simulink model "host_receive"  (R2015a)
settings: Solver=FixedStepDiscrete  StartTime=0.0  StopTime=inf  RelTol=1e-3
libraries: embdlinuxlib x2, simulink x1
settings Model: Creator=sbiagion  LastModifiedBy=sbiagion
settings DebuggingCC: UnderspecifiedInitializationDetection=Classic  MergeDetectMultiDrivingBlocksExec=none  SolverPrmCheckMsg=warning  MultiTaskRateTransMsg=warning

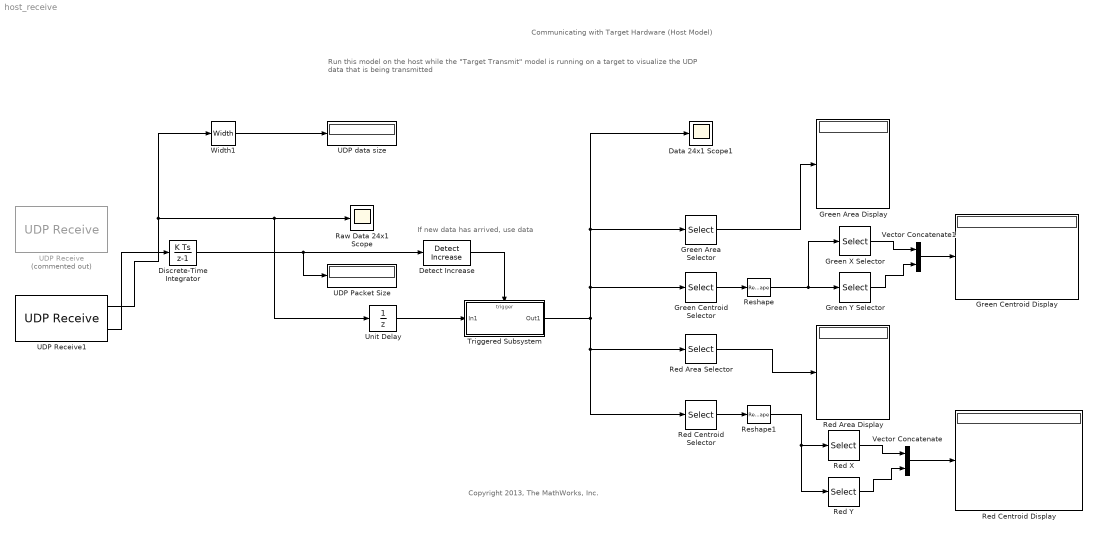
== system host_receive ==
  note: Run this model on the host while the "Target Transmit" model is running on a target to visualize the UDP data that is being transmitted
  note: Copyright 2013, The MathWorks, Inc.
  note: If new data has arrived, use data
  note: Communicating with Target Hardware
      | (Host Model)
  Data 24x1 Scope1 : Scope
      settings: ShowLegends=on  TimeRange=10  YMin=-100  YMax=1200  MaxDataPoints=100
  Detect Increase : simulink/Logic and Bit Operations/Detect Increase  vinit=0.0  InputProcessing=Inherited  OutDataTypeStr=boolean
  Discrete-Time Integrator : DiscreteIntegrator  gainval=1e4  SampleTime=-1
  Green Area Display : Display
  Green Area Selector : Selector  InputPortWidth=24  Indices=[1:4]
  Green Centroid Display : Display
  Green Centroid Selector : Selector  InputPortWidth=24  Indices=[5:12]
  Green X Selector : Selector  NumberOfDimensions=2  InputPortWidth=24  IndexOptions=Select all,Index vector (dialog)  Indices=[17:24],2  OutputSizes=1,1
  Green Y Selector : Selector  NumberOfDimensions=2  InputPortWidth=24  IndexOptions=Select all,Index vector (dialog)  Indices=[17:24],1  OutputSizes=1,1
  Raw Data 24x1 Scope : Scope
      settings: ShowLegends=on  TimeRange=10  YMin=-100  YMax=1200  MaxDataPoints=100
  Red Area Display : Display
  Red Area Selector : Selector  InputPortWidth=24  Indices=[13:16]
  Red Centroid Display : Display
  Red Centroid Selector : Selector  InputPortWidth=24  Indices=[17:24]
  Red X : Selector  NumberOfDimensions=2  InputPortWidth=24  IndexOptions=Select all,Index vector (dialog)  Indices=[17:24],2  OutputSizes=1,1
  Red Y : Selector  NumberOfDimensions=2  InputPortWidth=24  IndexOptions=Select all,Index vector (dialog)  Indices=[17:24],1  OutputSizes=1,1
  Reshape : Reshape  OutputDimensionality=Customize  OutputDimensions=[4,2]
  Reshape1 : Reshape  OutputDimensionality=Customize  OutputDimensions=[4,2]
  Triggered Subsystem : Subsystem  TreatAsAtomicUnit=on
  UDP Packet Size : Display
  UDP Receive : embdlinuxlib/UDP Receive  Commented=on  localURL='0.0.0.0'  localPort=25001  remoteURL='0.0.0.0'  remotePort=-1  recvBufferSize=8192  signalDatatype=int32  dims=24  isVarSize=off  showBlockingTime=off  blockingTime=0  sampletime=0.1  blockPlatform=BeagleBoard
  UDP Receive1 : embdlinuxlib/UDP Receive  localURL='0.0.0.0'  localPort=25000  remoteURL='0.0.0.0'  remotePort=-1  recvBufferSize=8192  signalDatatype=int32  dims=24  isVarSize=off  showBlockingTime=off  blockingTime=0  sampletime=0.1  blockPlatform=Raspberry Pi
  UDP data size : Display
  Unit Delay : UnitDelay  SampleTime=-1
  Vector Concatenate : Concatenate  Mode=Multidimensional array  ConcatenateDimension=2
  Vector Concatenate1 : Concatenate  Mode=Multidimensional array  ConcatenateDimension=2
  Width1 : Width
  wires:
  UDP Receive1/2 -> Discrete-Time Integrator/1
  Discrete-Time Integrator/1 -> UDP Packet Size/1, Detect Increase/1
  UDP Receive1/1 -> Width1/1, Unit Delay/1, Raw Data 24x1 Scope/1
  Width1/1 -> UDP data size/1
  Triggered Subsystem/1(Out1) -> Red Area Selector/1, Red Centroid Selector/1, Green Centroid Selector/1, Data 24x1 Scope1/1, Green Area Selector/1
  Detect Increase/1 -> Triggered Subsystem/Trigger
  Unit Delay/1 -> Triggered Subsystem/1(In1)
  Green Centroid Selector/1 -> Reshape/1
  Green Area Selector/1 -> Green Area Display/1
  Red Area Selector/1 -> Red Area Display/1
  Red Centroid Selector/1 -> Reshape1/1
  Reshape1/1 -> Red Y/1, Red X/1
  Red X/1 -> Vector Concatenate/1
  Red Y/1 -> Vector Concatenate/2
  Vector Concatenate/1 -> Red Centroid Display/1
  Reshape/1 -> Green X Selector/1, Green Y Selector/1
  Green X Selector/1 -> Vector Concatenate1/1
  Green Y Selector/1 -> Vector Concatenate1/2
  Vector Concatenate1/1 -> Green Centroid Display/1

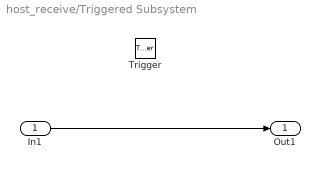
== system host_receive/Triggered Subsystem ==
  In1 : Inport
  Trigger : TriggerPort
  Out1 : Outport
  wires:
  In1/1 -> Out1/1
